simulink model "adc_ut"  (Simulink 8.1)
settings: Solver=FixedStepDiscrete  StartTime=0.0  StopTime=10.0  FixedStep=5E-3  RelTol=1e-3
libraries: siltestlib x6, adc x1
settings Model: Creator=AT015086  LastModifiedBy=tescamilla
settings DataIOCC: SignalLoggingSaveFormat=Dataset
settings OptimizationCC: ExpressionDepthLimit=128
settings DebuggingCC: FcnCallInpInsideContextMsg=EnableAllAsError
settings GRTTargetCC: CombineOutputUpdateFcns=on  GRTInterface=off

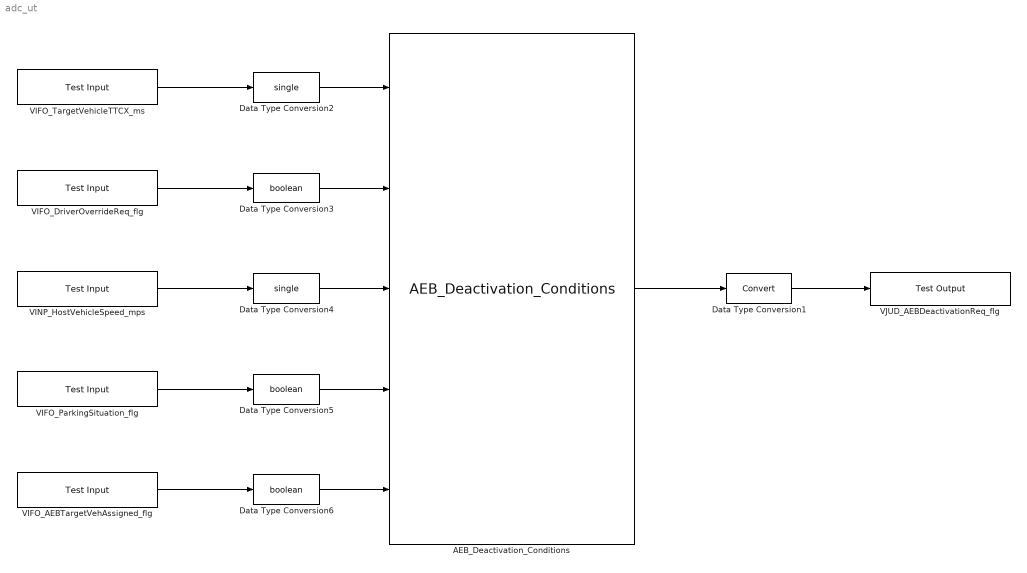
== system adc_ut ==
  AEB_Deactivation_Conditions : adc/AEB_Deactivation_Conditions
  Data Type Conversion1 : DataTypeConversion
  Data Type Conversion2 : DataTypeConversion  OutDataTypeStr=single
  Data Type Conversion3 : DataTypeConversion  OutDataTypeStr=boolean
  Data Type Conversion4 : DataTypeConversion  OutDataTypeStr=single
  Data Type Conversion5 : DataTypeConversion  OutDataTypeStr=boolean
  Data Type Conversion6 : DataTypeConversion  OutDataTypeStr=boolean
  VIFO_AEBTargetVehAssigned_flg : siltestlib/Test Input  varname=VIFO_AEBTargetVehAssigned_flg  sampletime=-1
  VIFO_DriverOverrideReq_flg : siltestlib/Test Input  varname=VIFO_DriverOverrideReq_flg  sampletime=-1
  VIFO_ParkingSituation_flg : siltestlib/Test Input  varname=VIFO_ParkingSituation_flg  sampletime=-1
  VIFO_TargetVehicleTTCX_ms : siltestlib/Test Input  varname=VIFO_TargetVehicleTTCX_ms  sampletime=-1
  VINP_HostVehicleSpeed_mps : siltestlib/Test Input  varname=VINP_HostVehicleSpeedA_mps  sampletime=-1
  VJUD_AEBDeactivationReq_flg : siltestlib/Test Output  varname=VJUD_AEBDeactivationReq_flg  sampletime=-1
  wires:
  AEB_Deactivation_Conditions/1 -> Data Type Conversion1/1
  Data Type Conversion1/1 -> VJUD_AEBDeactivationReq_flg/1
  VIFO_TargetVehicleTTCX_ms/1 -> Data Type Conversion2/1
  VIFO_DriverOverrideReq_flg/1 -> Data Type Conversion3/1
  VINP_HostVehicleSpeed_mps/1 -> Data Type Conversion4/1
  VIFO_ParkingSituation_flg/1 -> Data Type Conversion5/1
  VIFO_AEBTargetVehAssigned_flg/1 -> Data Type Conversion6/1
  Data Type Conversion2/1 -> AEB_Deactivation_Conditions/1
  Data Type Conversion3/1 -> AEB_Deactivation_Conditions/2
  Data Type Conversion4/1 -> AEB_Deactivation_Conditions/3
  Data Type Conversion5/1 -> AEB_Deactivation_Conditions/4
  Data Type Conversion6/1 -> AEB_Deactivation_Conditions/5
